simulink model "modelDE"  (R2019b)
settings: Solver=ode45  StartTime=0.0  StopTime=5  MaxStep=0.001  RelTol=1e-3
undefined symbols (not defined in the file): alfa, beta, c1, c2, J2, K, Tn
libraries: simulink_extras x2, simulink x1
settings Model: Creator=Mark  LastModifiedBy=Mark

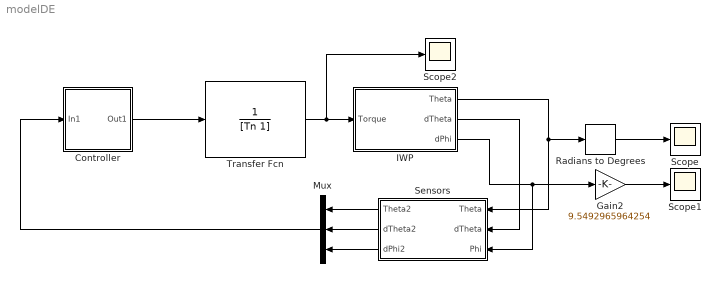
== system modelDE ==
  Controller : Subsystem  TreatAsAtomicUnit=on  SystemSampleTime=1/1000
  Gain2 : Gain  Gain=9.5492965964254
  IWP : Subsystem
  Mux : Mux  Inputs=3
  Radians to Degrees : simulink_extras/Transformations/Radians to Degrees
  Scope : Scope
  Scope1 : Scope
  Scope2 : Scope
  Sensors : Subsystem
  Transfer Fcn : TransferFcn  Denominator=[Tn 1]
  wires:
  IWP/1(Theta) -> Sensors/1(Theta), Radians to Degrees/1
  IWP/2(dTheta) -> Sensors/2(dTheta)
  IWP/3(dPhi) -> Sensors/3(Phi), Gain2/1
  Radians to Degrees/1 -> Scope/1
  Sensors/1(Theta2) -> Mux/1
  Sensors/2(dTheta2) -> Mux/2
  Sensors/3(dPhi2) -> Mux/3
  Gain2/1 -> Scope1/1
  Transfer Fcn/1 -> IWP/1(Torque), Scope2/1
  Mux/1 -> Controller/1(In1)
  Controller/1(Out1) -> Transfer Fcn/1

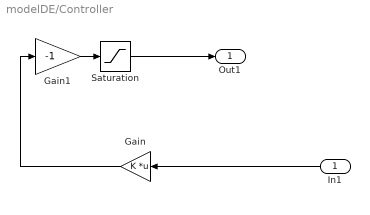
== system modelDE/Controller ==
  In1 : Inport
  Gain : Gain  Gain=K  Multiplication=Matrix(K*u)
  Gain1 : Gain  Gain=-1
  Saturation : Saturate
  Out1 : Outport
  wires:
  Gain1/1 -> Saturation/1
  Gain/1 -> Gain1/1
  Saturation/1 -> Out1/1
  In1/1 -> Gain/1

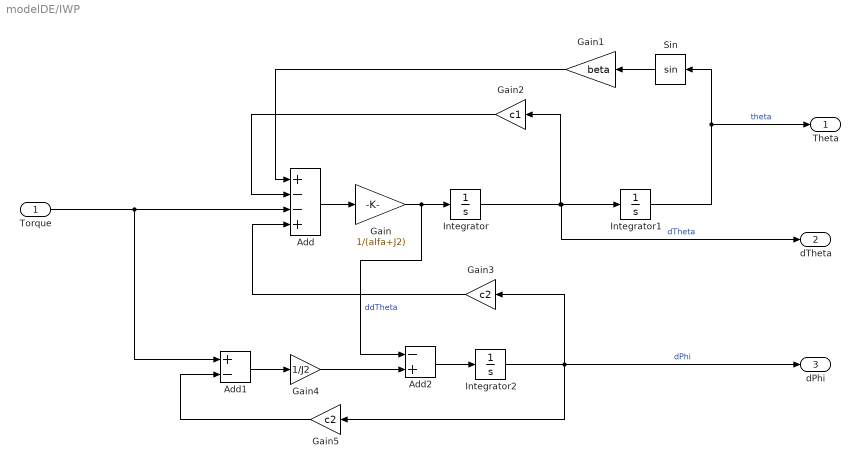
== system modelDE/IWP ==
  Torque : Inport
  Add : Sum  Inputs=+--+
  Add1 : Sum  Inputs=+-
  Add2 : Sum  Inputs=-+
  Gain : Gain  Gain=1/(alfa+J2)
  Gain1 : Gain  Gain=beta
  Gain2 : Gain  Gain=c1
  Gain3 : Gain  Gain=c2
  Gain4 : Gain  Gain=1/J2
  Gain5 : Gain  Gain=c2
  Integrator : Integrator
  Integrator1 : Integrator  InitialCondition=deg2rad(-3)
  Integrator2 : Integrator
  Sin : Trigonometry
  Theta : Outport
  dTheta : Outport  Port=2
  dPhi : Outport  Port=3
  wires:
  Gain1/1 -> Add/1
  Integrator1/1 -> Sin/1, Theta/1  "theta"
  Integrator2/1 -> Gain3/1, dPhi/1, Gain5/1  "dPhi"
  Integrator/1 -> Gain2/1, dTheta/1, Integrator1/1  "dTheta"
  Add1/1 -> Gain4/1
  Add2/1 -> Integrator2/1
  Gain5/1 -> Add1/2
  Torque/1 -> Add1/1, Add/3
  Gain3/1 -> Add/4
  Gain4/1 -> Add2/2
  Gain/1 -> Add2/1, Integrator/1  "ddTheta"
  Add/1 -> Gain/1
  Gain2/1 -> Add/2
  Sin/1 -> Gain1/1

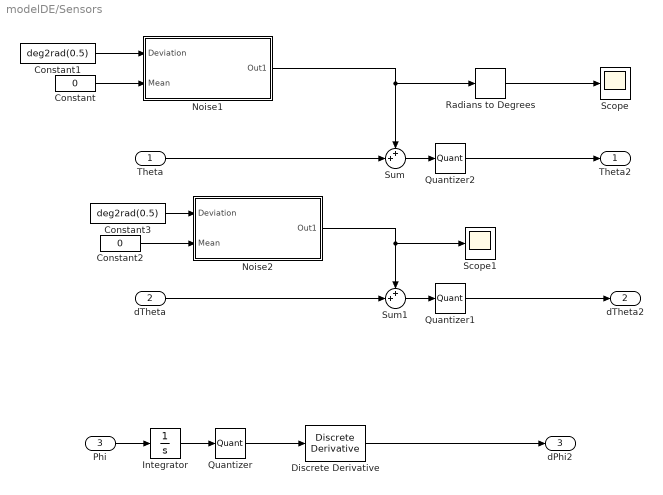
== system modelDE/Sensors ==
  Theta : Inport
  dTheta : Inport  Port=2
  Phi : Inport  Port=3
  Constant : Constant  Value=0
  Constant1 : Constant  Value=deg2rad(0.5)
  Constant2 : Constant  Value=0
  Constant3 : Constant  Value=deg2rad(0.5)
  Discrete Derivative : simulink/Discrete/Discrete Derivative  gainval=1.0  ICPrevScaledInput=0.0  OutMin=[]  OutMax=[]  OutDataType=fixdt(1, 16)  OutScaling=2^-10  DoSatur=off
  Integrator : Integrator
  Noise1 : Subsystem
  Noise2 : Subsystem
  Quantizer : Quantizer  QuantizationInterval=0.00001
  Quantizer1 : Quantizer  QuantizationInterval=0.00001
  Quantizer2 : Quantizer  QuantizationInterval=0.00001
  Radians to Degrees : simulink_extras/Transformations/Radians to Degrees
  Scope : Scope
  Scope1 : Scope
  Sum : Sum  Inputs=++|
  Sum1 : Sum  Inputs=++|
  Theta2 : Outport
  dTheta2 : Outport  Port=2
  dPhi2 : Outport  Port=3
  wires:
  Theta/1 -> Sum/2
  dTheta/1 -> Sum1/2
  Phi/1 -> Integrator/1
  Constant1/1 -> Noise1/1(Deviation)
  Constant/1 -> Noise1/2(Mean)
  Sum/1 -> Quantizer2/1
  Noise1/1(Out1) -> Sum/1, Radians to Degrees/1
  Constant3/1 -> Noise2/1(Deviation)
  Constant2/1 -> Noise2/2(Mean)
  Sum1/1 -> Quantizer1/1
  Noise2/1(Out1) -> Scope1/1, Sum1/1
  Quantizer/1 -> Discrete Derivative/1
  Radians to Degrees/1 -> Scope/1
  Discrete Derivative/1 -> dPhi2/1
  Integrator/1 -> Quantizer/1
  Quantizer2/1 -> Theta2/1
  Quantizer1/1 -> dTheta2/1

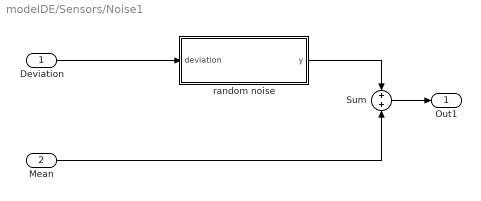
== system modelDE/Sensors/Noise1 ==
  Deviation : Inport
  Mean : Inport  Port=2
  Sum : Sum
  random noise : MATLAB Function  TreatAsAtomicUnit=on  SystemSampleTime=0.001
  Out1 : Outport
  wires:
  Deviation/1 -> random noise/1(deviation)
  random noise/1(y) -> Sum/1
  Mean/1 -> Sum/2
  Sum/1 -> Out1/1

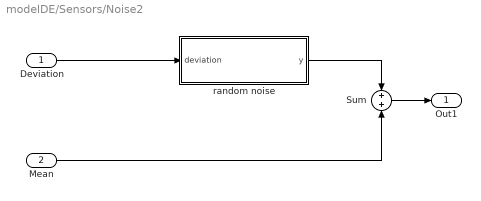
== system modelDE/Sensors/Noise2 ==
  Deviation : Inport
  Mean : Inport  Port=2
  Sum : Sum
  random noise : MATLAB Function  TreatAsAtomicUnit=on  SystemSampleTime=0.001
  Out1 : Outport
  wires:
  Deviation/1 -> random noise/1(deviation)
  random noise/1(y) -> Sum/1
  Mean/1 -> Sum/2
  Sum/1 -> Out1/1

== matlab function modelDE/Sensors/Noise2/random noise ==
  data: y output; deviation input
function y = fcn(deviation)

y = (deviation*randn());

== matlab function modelDE/Sensors/Noise1/random noise ==
  data: y output; deviation input
function y = fcn(deviation)

y = (deviation*randn());
